simulink model "selector"  (R2020a)
settings: Solver=VariableStepAuto  StartTime=0.0  StopTime=inf  RelTol=1e-3
settings Model: Creator=F1  LastModifiedBy=F1

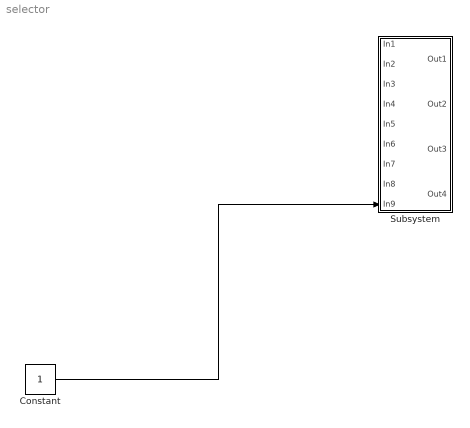
== system selector ==
  Constant : Constant
  Subsystem : Subsystem
  wires:
  Constant/1 -> Subsystem/9(In9)

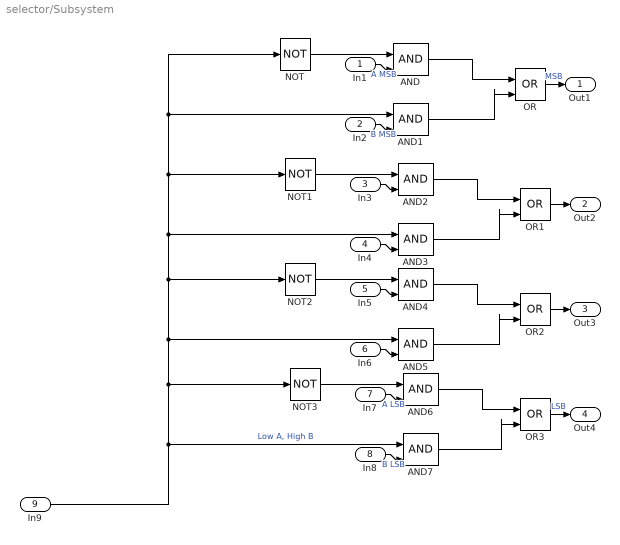
== system selector/Subsystem ==
  In1 : Inport
  In2 : Inport  Port=2
  In3 : Inport  Port=3
  In4 : Inport  Port=4
  In5 : Inport  Port=5
  In6 : Inport  Port=6
  In7 : Inport  Port=7
  In8 : Inport  Port=8
  In9 : Inport  Port=9
  AND{,1..7} (8 alike) : Logic  IconShape=distinctive  AllPortsSameDT=off  OutDataTypeStr=boolean
  NOT{,1..3} (4 alike) : Logic  Operator=NOT  IconShape=distinctive  AllPortsSameDT=off  OutDataTypeStr=boolean
  OR{,1..3} (4 alike) : Logic  Operator=OR  IconShape=distinctive  AllPortsSameDT=off  OutDataTypeStr=boolean
  Out1 : Outport
  Out2 : Outport  Port=2
  Out3 : Outport  Port=3
  Out4 : Outport  Port=4
  wires:
  In9/1 -> AND7/1, NOT3/1, AND5/1, NOT2/1, NOT1/1, AND1/1, NOT/1, AND3/1  "Low A, High B"
  AND5/1 -> OR2/2
  NOT/1 -> AND/1
  NOT1/1 -> AND2/1
  AND/1 -> OR/1
  AND2/1 -> OR1/1
  In4/1 -> AND3/2
  NOT2/1 -> AND4/1
  AND3/1 -> OR1/2
  AND4/1 -> OR2/1
  OR1/1 -> Out2/1
  In5/1 -> AND4/2
  AND7/1 -> OR3/2
  AND1/1 -> OR/2
  OR/1 -> Out1/1  "MSB"
  AND6/1 -> OR3/1
  In3/1 -> AND2/2
  OR2/1 -> Out3/1
  NOT3/1 -> AND6/1
  In2/1 -> AND1/2  "B MSB"
  In6/1 -> AND5/2
  In1/1 -> AND/2  "A MSB"
  In8/1 -> AND7/2  "B LSB"
  In7/1 -> AND6/2  "A LSB"
  OR3/1 -> Out4/1  "LSB"
